simulink model "second_2"  (R2022b)
settings: Solver=VariableStepAuto  StartTime=0.0  StopTime=200  FixedStep=0.001  RelTol=1e-3
values from neighbouring files (symbols this model uses):
  a = ab(1)    [dyskretny_skrypt2.m]
  b = ab(2)    [dyskretny_skrypt2.m]
settings Model: Creator=zuzanna  LastModifiedBy=zuzanna

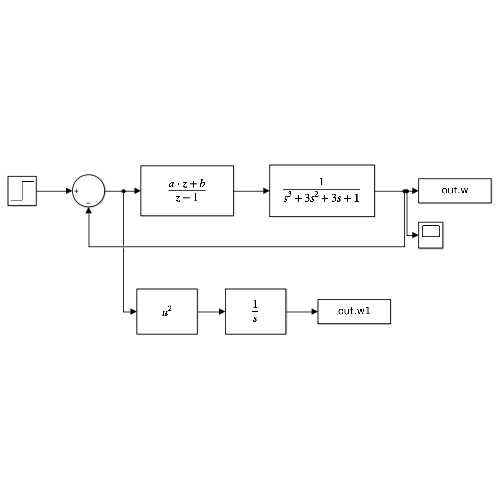
[thumbnail: Simulink's stored preview of the top-level diagram]
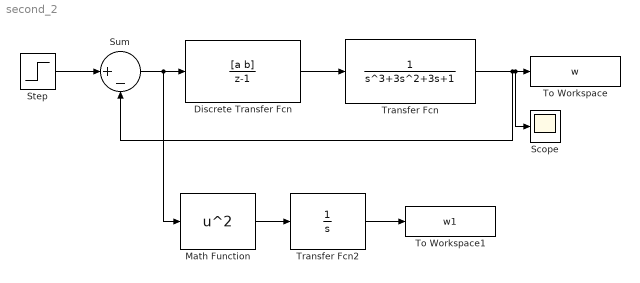
== system second_2 ==
  Discrete Transfer Fcn : DiscreteTransferFcn  Numerator=[a b]  Denominator=[1 -1]  SampleTime=1
  Math Function : Math  Operator=square
  Scope : Scope
  Step : Step  SampleTime=0
  Sum : Sum  Inputs=|+-
  To Workspace : ToWorkspace  VariableName=w  SampleTime=-1
  To Workspace1 : ToWorkspace  VariableName=w1  SampleTime=-1
  Transfer Fcn : TransferFcn  Denominator=[1 3 3 1]
  Transfer Fcn2 : TransferFcn  Denominator=[1 0]
  wires:
  Transfer Fcn/1 -> Scope/1, To Workspace/1, Sum/2
  Discrete Transfer Fcn/1 -> Transfer Fcn/1
  Sum/1 -> Math Function/1, Discrete Transfer Fcn/1
  Step/1 -> Sum/1
  Math Function/1 -> Transfer Fcn2/1
  Transfer Fcn2/1 -> To Workspace1/1
